simulink model "k1visproto"  (Simulink 8.2)
settings: Solver=ode45  StartTime=0.0  StopTime=10.0  RelTol=1e-3
libraries: cdsFiltCtrl x82, cdsFilt x45, cdsMuxMatrix x18, cdsEpicsOut x7, cdsEpicsBinIn x2, cdsAdcx0 x1, cdsAdcx1 x1, dac x1, simulink x1, cdsParameters x1
(part 6 of 14)

== system k1visproto/PROTO/GAS/SERVOF ==
  F0_IN : Inport
  F1_IN : Inport  Port=2
  F2_IN : Inport  Port=3
  F0 : cdsFiltCtrl/IIR FM with control  Tag=cdsFiltCtrl  Description=|
      | cdsFiltCntrl is the standard IIR filter module (exactly the same as cdsFilt) but with added control data output 'Ctrl'. Filter module digital signal output appears on the first output, which is called 'Val'. 'Ctrl' output has a bit pattern encoding the state of filter's on/off switches (FM1 through FM10). The bit values are:
      |                                                                                                                                                                                                                                                                                                                                       
      | module 	hex	dec                                                                                                                                                                                                                                                                                                                       
      | -----------------------                                                                                                                                                                                                                                                                                                               
      | FM1	0x20                    32                                                                                                                                                                                                                                                                                                        
      | FM2	0x80                     128                                                                                                                                                                                                                                                                                                      
      | FM3	0x200                   512                                                                                                                                                                                                                                                                                                       
      | FM4	0x800                   2048                                                                                                                                                                                                                                                                                                      
      | FM5	0x2000                 8192                                                                                                                                                                                                                                                                                                       
      | FM6	0x8000                 32768                                                                                                                                                                                                                                                                                                      
      | FM7	0x20000                131072                                                                                                                                                                                                                                                                                                     
      | FM8	0x80000                 524288                                                                                                                                                                                                                                                                                                    
      | FM9	0x200000               2097152                                                                                                                                                                                                                                                                                                    
      | FM10	0x800000               8388608                                                                                                                                                                                                                                                                                                   
      |                                                                                                                                                                                                                                                                                                                                       
      | This bit data can be used to drive some other switches or it can be output using a binary I/O module.
      settings: AttributesFormatString=%<Tag>
  F1 : cdsFiltCtrl/IIR FM with control  Tag=cdsFiltCtrl  Description=|
      | cdsFiltCntrl is the standard IIR filter module (exactly the same as cdsFilt) but with added control data output 'Ctrl'. Filter module digital signal output appears on the first output, which is called 'Val'. 'Ctrl' output has a bit pattern encoding the state of filter's on/off switches (FM1 through FM10). The bit values are:
      |                                                                                                                                                                                                                                                                                                                                       
      | module 	hex	dec                                                                                                                                                                                                                                                                                                                       
      | -----------------------                                                                                                                                                                                                                                                                                                               
      | FM1	0x20                    32                                                                                                                                                                                                                                                                                                        
      | FM2	0x80                     128                                                                                                                                                                                                                                                                                                      
      | FM3	0x200                   512                                                                                                                                                                                                                                                                                                       
      | FM4	0x800                   2048                                                                                                                                                                                                                                                                                                      
      | FM5	0x2000                 8192                                                                                                                                                                                                                                                                                                       
      | FM6	0x8000                 32768                                                                                                                                                                                                                                                                                                      
      | FM7	0x20000                131072                                                                                                                                                                                                                                                                                                     
      | FM8	0x80000                 524288                                                                                                                                                                                                                                                                                                    
      | FM9	0x200000               2097152                                                                                                                                                                                                                                                                                                    
      | FM10	0x800000               8388608                                                                                                                                                                                                                                                                                                   
      |                                                                                                                                                                                                                                                                                                                                       
      | This bit data can be used to drive some other switches or it can be output using a binary I/O module.
      settings: AttributesFormatString=%<Tag>
  F2 : cdsFiltCtrl/IIR FM with control  Tag=cdsFiltCtrl  Description=|
      | cdsFiltCntrl is the standard IIR filter module (exactly the same as cdsFilt) but with added control data output 'Ctrl'. Filter module digital signal output appears on the first output, which is called 'Val'. 'Ctrl' output has a bit pattern encoding the state of filter's on/off switches (FM1 through FM10). The bit values are:
      |                                                                                                                                                                                                                                                                                                                                       
      | module 	hex	dec                                                                                                                                                                                                                                                                                                                       
      | -----------------------                                                                                                                                                                                                                                                                                                               
      | FM1	0x20                    32                                                                                                                                                                                                                                                                                                        
      | FM2	0x80                     128                                                                                                                                                                                                                                                                                                      
      | FM3	0x200                   512                                                                                                                                                                                                                                                                                                       
      | FM4	0x800                   2048                                                                                                                                                                                                                                                                                                      
      | FM5	0x2000                 8192                                                                                                                                                                                                                                                                                                       
      | FM6	0x8000                 32768                                                                                                                                                                                                                                                                                                      
      | FM7	0x20000                131072                                                                                                                                                                                                                                                                                                     
      | FM8	0x80000                 524288                                                                                                                                                                                                                                                                                                    
      | FM9	0x200000               2097152                                                                                                                                                                                                                                                                                                    
      | FM10	0x800000               8388608                                                                                                                                                                                                                                                                                                   
      |                                                                                                                                                                                                                                                                                                                                       
      | This bit data can be used to drive some other switches or it can be output using a binary I/O module.
      settings: AttributesFormatString=%<Tag>
  Ground1 : Ground
  Ground2 : Ground
  Ground3 : Ground
  Terminator1 : Terminator
  Terminator2 : Terminator
  Terminator3 : Terminator
  F0_Out : Outport
  F1_Out : Outport  Port=2
  F2_Out : Outport  Port=3
  wires:
  F0/2 -> Terminator1/1
  Ground1/1 -> F0/2
  F0_IN/1 -> F0/1
  F1/2 -> Terminator2/1
  Ground2/1 -> F1/2
  F1_IN/1 -> F1/1
  F2/2 -> Terminator3/1
  Ground3/1 -> F2/2
  F2_IN/1 -> F2/1
  F0/1 -> F0_Out/1
  F1/1 -> F1_Out/1
  F2/1 -> F2_Out/1

== system k1visproto/PROTO/GAS/TEST ==
  F0 : cdsFilt/Subsystem  Tag=cdsFilt  Description=|
      | Purpose:                                                                                                                                                                                                                                  
      | Standard CDS IIR filter module.                                                                                                                                                                                                           
      |                                                                                                                                                                                                                                           
      | Operation:                                                                                                                                                                                                                                
      | Consists of 10 second order section IIR filters, plus a ramped gain stage. In FE code, also provides pre-defined test points and excitation channel inputs. The filter coefficients are defined in the LIGO system using the 'foton' tool.
      |                                                                                                                                                                                                                                           
      | Usage:                                                                                                                                                                                                                                    
      | Name the part with the desired filter module name.
      settings: AttributesFormatString=%<Tag>
  F1 : cdsFilt/Subsystem  Tag=cdsFilt  Description=|
      | Purpose:                                                                                                                                                                                                                                  
      | Standard CDS IIR filter module.                                                                                                                                                                                                           
      |                                                                                                                                                                                                                                           
      | Operation:                                                                                                                                                                                                                                
      | Consists of 10 second order section IIR filters, plus a ramped gain stage. In FE code, also provides pre-defined test points and excitation channel inputs. The filter coefficients are defined in the LIGO system using the 'foton' tool.
      |                                                                                                                                                                                                                                           
      | Usage:                                                                                                                                                                                                                                    
      | Name the part with the desired filter module name.
      settings: AttributesFormatString=%<Tag>
  F2 : cdsFilt/Subsystem  Tag=cdsFilt  Description=|
      | Purpose:                                                                                                                                                                                                                                  
      | Standard CDS IIR filter module.                                                                                                                                                                                                           
      |                                                                                                                                                                                                                                           
      | Operation:                                                                                                                                                                                                                                
      | Consists of 10 second order section IIR filters, plus a ramped gain stage. In FE code, also provides pre-defined test points and excitation channel inputs. The filter coefficients are defined in the LIGO system using the 'foton' tool.
      |                                                                                                                                                                                                                                           
      | Usage:                                                                                                                                                                                                                                    
      | Name the part with the desired filter module name.
      settings: AttributesFormatString=%<Tag>
  Ground1 : Ground
  Ground2 : Ground
  Ground3 : Ground
  F0_Out : Outport
  F1_Out : Outport  Port=2
  F2_Out : Outport  Port=3
  wires:
  F2/1 -> F2_Out/1
  F1/1 -> F1_Out/1
  F0/1 -> F0_Out/1
  Ground1/1 -> F0/1
  Ground2/1 -> F1/1
  Ground3/1 -> F2/1

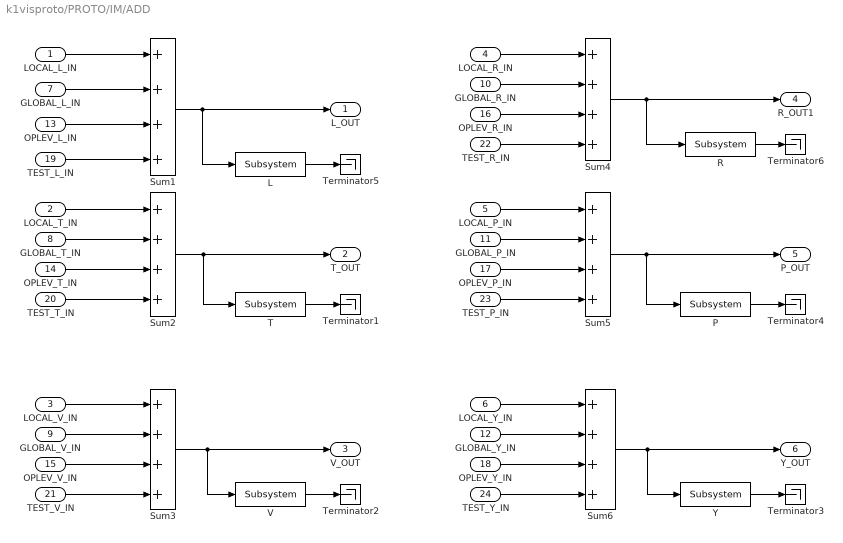
== system k1visproto/PROTO/IM/ADD ==
  LOCAL_L_IN : Inport
  LOCAL_T_IN : Inport  Port=2
  LOCAL_V_IN : Inport  Port=3
  LOCAL_R_IN : Inport  Port=4
  LOCAL_P_IN : Inport  Port=5
  LOCAL_Y_IN : Inport  Port=6
  GLOBAL_L_IN : Inport  Port=7
  GLOBAL_T_IN : Inport  Port=8
  GLOBAL_V_IN : Inport  Port=9
  GLOBAL_R_IN : Inport  Port=10
  GLOBAL_P_IN : Inport  Port=11
  GLOBAL_Y_IN : Inport  Port=12
  OPLEV_L_IN : Inport  Port=13
  OPLEV_T_IN : Inport  Port=14
  OPLEV_V_IN : Inport  Port=15
  OPLEV_R_IN : Inport  Port=16
  OPLEV_P_IN : Inport  Port=17
  OPLEV_Y_IN : Inport  Port=18
  TEST_L_IN : Inport  Port=19
  TEST_T_IN : Inport  Port=20
  TEST_V_IN : Inport  Port=21
  TEST_R_IN : Inport  Port=22
  TEST_P_IN : Inport  Port=23
  TEST_Y_IN : Inport  Port=24
  L : cdsFilt/Subsystem  Tag=cdsFilt  Description=|
      | Purpose:                                                                                                                                                                                                                                  
      | Standard CDS IIR filter module.                                                                                                                                                                                                           
      |                                                                                                                                                                                                                                           
      | Operation:                                                                                                                                                                                                                                
      | Consists of 10 second order section IIR filters, plus a ramped gain stage. In FE code, also provides pre-defined test points and excitation channel inputs. The filter coefficients are defined in the LIGO system using the 'foton' tool.
      |                                                                                                                                                                                                                                           
      | Usage:                                                                                                                                                                                                                                    
      | Name the part with the desired filter module name.
      settings: AttributesFormatString=%<Tag>
  P : cdsFilt/Subsystem  Tag=cdsFilt  Description=|
      | Purpose:                                                                                                                                                                                                                                  
      | Standard CDS IIR filter module.                                                                                                                                                                                                           
      |                                                                                                                                                                                                                                           
      | Operation:                                                                                                                                                                                                                                
      | Consists of 10 second order section IIR filters, plus a ramped gain stage. In FE code, also provides pre-defined test points and excitation channel inputs. The filter coefficients are defined in the LIGO system using the 'foton' tool.
      |                                                                                                                                                                                                                                           
      | Usage:                                                                                                                                                                                                                                    
      | Name the part with the desired filter module name.
      settings: AttributesFormatString=%<Tag>
  R : cdsFilt/Subsystem  Tag=cdsFilt  Description=|
      | Purpose:                                                                                                                                                                                                                                  
      | Standard CDS IIR filter module.                                                                                                                                                                                                           
      |                                                                                                                                                                                                                                           
      | Operation:                                                                                                                                                                                                                                
      | Consists of 10 second order section IIR filters, plus a ramped gain stage. In FE code, also provides pre-defined test points and excitation channel inputs. The filter coefficients are defined in the LIGO system using the 'foton' tool.
      |                                                                                                                                                                                                                                           
      | Usage:                                                                                                                                                                                                                                    
      | Name the part with the desired filter module name.
      settings: AttributesFormatString=%<Tag>
  Sum{1..6} (6 alike) : Sum  Inputs=++++
  T : cdsFilt/Subsystem  Tag=cdsFilt  Description=|
      | Purpose:                                                                                                                                                                                                                                  
      | Standard CDS IIR filter module.                                                                                                                                                                                                           
      |                                                                                                                                                                                                                                           
      | Operation:                                                                                                                                                                                                                                
      | Consists of 10 second order section IIR filters, plus a ramped gain stage. In FE code, also provides pre-defined test points and excitation channel inputs. The filter coefficients are defined in the LIGO system using the 'foton' tool.
      |                                                                                                                                                                                                                                           
      | Usage:                                                                                                                                                                                                                                    
      | Name the part with the desired filter module name.
      settings: AttributesFormatString=%<Tag>
  Terminator{1..6} (6 alike) : Terminator
  V : cdsFilt/Subsystem  Tag=cdsFilt  Description=|
      | Purpose:                                                                                                                                                                                                                                  
      | Standard CDS IIR filter module.                                                                                                                                                                                                           
      |                                                                                                                                                                                                                                           
      | Operation:                                                                                                                                                                                                                                
      | Consists of 10 second order section IIR filters, plus a ramped gain stage. In FE code, also provides pre-defined test points and excitation channel inputs. The filter coefficients are defined in the LIGO system using the 'foton' tool.
      |                                                                                                                                                                                                                                           
      | Usage:                                                                                                                                                                                                                                    
      | Name the part with the desired filter module name.
      settings: AttributesFormatString=%<Tag>
  Y : cdsFilt/Subsystem  Tag=cdsFilt  Description=|
      | Purpose:                                                                                                                                                                                                                                  
      | Standard CDS IIR filter module.                                                                                                                                                                                                           
      |                                                                                                                                                                                                                                           
      | Operation:                                                                                                                                                                                                                                
      | Consists of 10 second order section IIR filters, plus a ramped gain stage. In FE code, also provides pre-defined test points and excitation channel inputs. The filter coefficients are defined in the LIGO system using the 'foton' tool.
      |                                                                                                                                                                                                                                           
      | Usage:                                                                                                                                                                                                                                    
      | Name the part with the desired filter module name.
      settings: AttributesFormatString=%<Tag>
  L_OUT : Outport
  T_OUT : Outport  Port=2
  V_OUT : Outport  Port=3
  R_OUT1 : Outport  Port=4
  P_OUT : Outport  Port=5
  Y_OUT : Outport  Port=6
  wires:
  GLOBAL_L_IN/1 -> Sum1/2
  LOCAL_T_IN/1 -> Sum2/1
  LOCAL_V_IN/1 -> Sum3/1
  LOCAL_L_IN/1 -> Sum1/1
  GLOBAL_P_IN/1 -> Sum5/2
  LOCAL_P_IN/1 -> Sum5/1
  LOCAL_Y_IN/1 -> Sum6/1
  LOCAL_R_IN/1 -> Sum4/1
  GLOBAL_Y_IN/1 -> Sum6/2
  TEST_P_IN/1 -> Sum5/4
  TEST_Y_IN/1 -> Sum6/4
  OPLEV_P_IN/1 -> Sum5/3
  OPLEV_Y_IN/1 -> Sum6/3
  Sum1/1 -> L/1, L_OUT/1
  Sum2/1 -> T/1, T_OUT/1
  Sum3/1 -> V/1, V_OUT/1
  Sum4/1 -> R_OUT1/1, R/1
  Sum5/1 -> P/1, P_OUT/1
  Sum6/1 -> Y/1, Y_OUT/1
  L/1 -> Terminator5/1
  T/1 -> Terminator1/1
  V/1 -> Terminator2/1
  Y/1 -> Terminator3/1
  P/1 -> Terminator4/1
  R/1 -> Terminator6/1
  TEST_T_IN/1 -> Sum2/4
  TEST_V_IN/1 -> Sum3/4
  OPLEV_L_IN/1 -> Sum1/3
  TEST_L_IN/1 -> Sum1/4
  TEST_R_IN/1 -> Sum4/4
  GLOBAL_R_IN/1 -> Sum4/2
  OPLEV_R_IN/1 -> Sum4/3
  GLOBAL_T_IN/1 -> Sum2/2
  OPLEV_T_IN/1 -> Sum2/3
  GLOBAL_V_IN/1 -> Sum3/2
  OPLEV_V_IN/1 -> Sum3/3

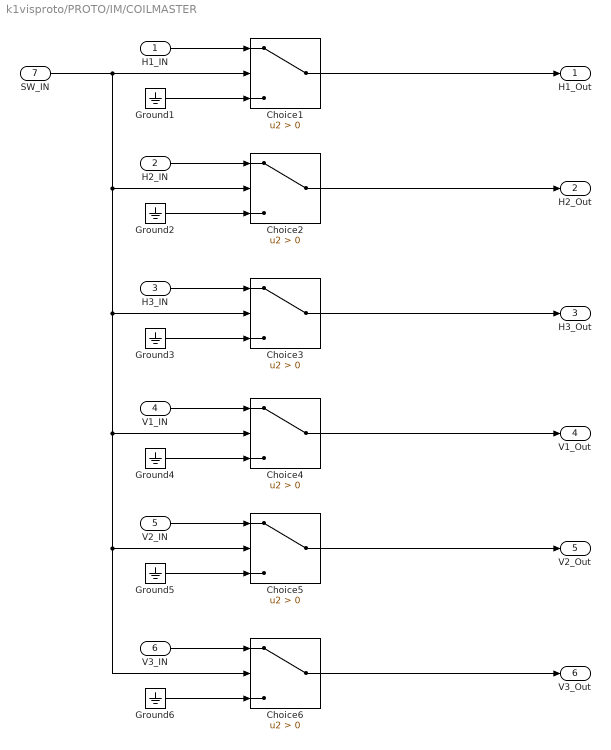
== system k1visproto/PROTO/IM/COILMASTER ==
  H1_IN : Inport
  H2_IN : Inport  Port=2
  H3_IN : Inport  Port=3
  V1_IN : Inport  Port=4
  V2_IN : Inport  Port=5
  V3_IN : Inport  Port=6
  SW_IN : Inport  Port=7
  Choice{1..6} (6 alike) : Switch  Criteria=u2 > Threshold
  Ground{1..6} (6 alike) : Ground
  H1_Out : Outport
  H2_Out : Outport  Port=2
  H3_Out : Outport  Port=3
  V1_Out : Outport  Port=4
  V2_Out : Outport  Port=5
  V3_Out : Outport  Port=6
  wires:
  Choice3/1 -> H3_Out/1
  Choice2/1 -> H2_Out/1
  Choice1/1 -> H1_Out/1
  SW_IN/1 -> Choice1/2, Choice6/2, Choice5/2, Choice4/2, Choice3/2, Choice2/2
  H3_IN/1 -> Choice3/1
  Ground3/1 -> Choice3/3
  Ground2/1 -> Choice2/3
  H2_IN/1 -> Choice2/1
  Ground1/1 -> Choice1/3
  H1_IN/1 -> Choice1/1
  Choice5/1 -> V2_Out/1
  Choice4/1 -> V1_Out/1
  Choice6/1 -> V3_Out/1
  V3_IN/1 -> Choice6/1
  Ground6/1 -> Choice6/3
  Ground5/1 -> Choice5/3
  V2_IN/1 -> Choice5/1
  Ground4/1 -> Choice4/3
  V1_IN/1 -> Choice4/1
